simulink model "test_quadcopter"  (R2021b)
settings: Solver=ode45  StartTime=0.0  StopTime=300  FixedStep=Ts  MaxStep=0.001  RelTol=1e-3  AbsTol=1e-3
model workspace (MATLAB code in the model file):
  | load('xy_data_membrane.mat');
undefined symbols (not defined in the file): kd_altitude, kd_attitude, kd_position, ki_altitude, ki_attitude, kp_altitude, kp_attitude, kp_position, propeller, X, x0, xrot, Y, y0, yrot, Z, z0, zrot
libraries: sm_lib x83, fl_lib x40, nesl_utility x34, aerolibwind2 x6, slpidlib x4
(part 1 of 4)
settings Model: Creator=The MathWorks, Inc.  LastModifiedBy=tejaswi
settings SolverCC: AutoScaleAbsTol=off  ZeroCrossAlgorithm=Adaptive  AlgebraicLoopSolver=TrustRegion  SolverResetMethod=Robust
settings DataIOCC: ReturnWorkspaceOutputs=off  SignalLoggingName=logsout_sm_quadcopter
settings DebuggingCC: IgnoredZcDiagnostic=none  SFMachineParentedDataDiag=warning
settings SimscapeCC: SimscapeLogType=all  SimscapeLogSimulationStatistics=on  SimscapeLogName=simlog_sm_quadcopter  SimscapeLogLimitData=off
settings DiagnosticsConfigSet: SimMechanicsRigidlyBoundBlock=none
settings ExplorerConfigSet: InternalSimMechanicsExplorerSettings="<ExplorerConfiguration><canonicalview>default</canonicalview><AnimationSetting><BasePlaybackSpeed>1.0</BasePlaybackSpeed><PlaybackSpeedFactor>1.0</PlaybackSpeedFactor></AnimationSetting><TilePanel><TileInfo><Tiles Columns=\"1\" Count=\"1\" Rows=\"1\"><Column Weight=\"1\"/><Row Weight=\"1\"/><Tile Height=\"1\" Width=\"1\" X=\"0\" Y=\"0\"/></Tiles></TileInfo><SceneInfo><SceneViewer><BGColor><R>0.400000005960464478</R><G>0.800000011920928955</G><B>1</B></BGColor><Camera><DoPerspective>on</DoPerspective><Position><X>-6.15419739613543015e-08</X><Y>-14.2688678910713858</Y><Z>-0.120593802588993895</Z></Position><Center><X>-6.15419739613543015e-08</X><Y>-5.00943414473349335</Y><Z>-0.120593802588992993</Z></Center><Up><X>0</X><Y>-2.49956154589103037e-16</Y><Z>1</Z></Up><ViewLimDist>1</ViewLimDist><YLim>0.466307658154998583</YLim><XLim>0.642537642675115039</XLim></Camera></SceneViewer></SceneInfo></TilePanel><MechEditorPanel><Cameras><Camera><Id>Camera1</Id><Value><Name>Camera1</Name><NativeCamera><PositionKeyframeSet><Keyframe><Time>0</Time><Value><X>-6.1541973961354302e-08</X><Y>-14.268867891071386</Y><Z>-0.1205938025889939</Z></Value></Keyframe><Keyframe><Time>1.9750000000000001</Time><Value><X>0.69357816146467988</X><Y>-14.804552995771699</Y><Z>2.1747680387120214</Z></Value></Keyframe><Keyframe><Time>4.0499999999999998</Time><Value><X>-1.6597740498874662</X><Y>-11.736154408489586</Y><Z>3.2279651603213511</Z></Value></Keyframe><Keyframe><Time>6</Time><Value><X>-1.4506804349012337</X><Y>-10.190737244494224</Y><Z>3.5728880702176977</Z></Value></Keyframe><Keyframe><Time>8</Time><Value><X>-1.6299263783474844</X><Y>-10.672186518254485</Y><Z>3.1366411391344338</Z></Value></Keyframe><Keyframe><Time>10</Time><Value><X>0.18587558187085493</X><Y>-7.6738882503163852</Y><Z>3.8257660713229682</Z></Value></Keyframe><Keyframe><Time>12</Time><Value><X>1.4883977802616708</X><Y>-8.4980171831454285</Y><Z>3.8627593448850166</Z></Value></Keyframe><Keyframe><Time>14</Time><Value><X>1.9893590360011646</X><Y>-6.4957785736357501</Y><Z>3.7251488250353217</Z></Value></Keyframe><Keyframe><Time>16</Time><Value><X>3.6270195589678793</X><Y>-6.36852658984645</Y><Z>3.5837326656674442</Z></Value></Keyframe><Keyframe><Time>18</Time><Value><X>4.1090510945125924</X><Y>-5.5357120217518236</Y><Z>3.2752105329973098</Z></Value></Keyframe><Keyframe><Time>20</Time><Value><X>4.1663622380806169</X><Y>-4.0387452486279827</Y><Z>2.5605170976103575</Z></Value></Keyframe><Keyframe><Time>22</Time><Value><X>4.859351912085474</X><Y>-0.43949351172743789</Y><Z>0.95256853851762346</Z></Value></Keyframe></PositionKeyframeSet><CenterKeyframeSet><Keyframe><Time>0</Time><Value><X>-6.1541973961354302e-08</X><Y>-5.0094341447334934</Y><Z>-0.12059380258899299</Z></Value></Keyframe><Keyframe><Time>1.9750000000000001</Time><Value><X>0.69348438643822474</X><Y>-5.2781774058054065</Y><Z>2.1823800390633106</Z></Value></Keyframe><Keyframe><Time>4.0499999999999998</Time><Value><X>-1.687564798021405</X><Y>-3.7348295538313101</Y><Z>3.2262958119221108</Z></Value></Keyframe><Keyframe><Time>6</Time><Value><X>-1.4797051298603214</X><Y>-2.960851752431255</Y><Z>3.5728880702177048</Z></Value></Keyframe><Keyframe><Time>8</Time><Value><X>-1.5997478000361871</X><Y>-3.1953029757138154</Y><Z>3.1365999604490469</Z></Value></Keyframe><Keyframe><Time>10</Time><Value><X>0.24405104343601497</X><Y>-1.6873776010017201</Y><Z>3.8387300040675179</Z></Value></Keyframe><Keyframe><Time>12</Time><Value><X>1.4806541700514058</X><Y>-2.1382106204808444</Y><Z>3.9209906203717133</Z></Value></Keyframe><Keyframe><Time>14</Time><Value><X>1.9523323695945445</X><Y>-1.1203987104972244</Y><Z>3.7938236446623668</Z></Value></Keyframe><Keyframe><Time>16</Time><Value><X>3.5048147463492194</X><Y>-0.99103496830061388</Y><Z>3.6957539225348288</Z></Value></Keyframe><Keyframe><Time>18</Time><Value><X>3.9997564750585872</X><Y>-0.58040744208225181</Y><Z>3.4078217139748177</Z></Value></Keyframe><Keyframe><Time>20</Time><Value><X>4.1020127201493066</X><Y>0.13918949483856302</Y><Z>2.6890918744946277</Z></Value></Keyframe><Keyframe><Time>22</Time><Value><X>4.822225130199671</X><Y>1.9709872026638768</Y><Z>1.0267504104392398</Z></Value></Keyframe></CenterKeyframeSet><UpVectorKeyframeSet><Keyframe><Time>0</Time><Value><X>0</X><Y>-2.4995615458910304e-16</Y><Z>1</Z></Value></Keyframe><Keyframe><Time>1.9750000000000001</Time><Value><X>7.8655746289375513e-09</X><Y>-0.00079904448954799042</Y><Z>0.99999968076390089</Z></Value></Keyframe><Keyframe><Time>4.0499999999999998</Time><Value><X>-7.2455634795717249e-07</X><Y>0.00020863147757072589</Y><Z>0.99999997823619069</Z></Value></Keyframe><Keyframe><Time>6</Time><Value><X>1.915739347589952e-18</X><Y>-4.771997133902034e-16</Y><Z>1</Z></Value></Keyframe><Keyframe><Time>8</Time><Value><X>-9.4628750535966929e-06</X><Y>5.5456610049874724e-06</Y><Z>0.99999999993984978</Z></Value></Keyframe><Keyframe><Time>10</Time><Value><X>-2.1042002088428629e-05</X><Y>-0.002165314484770997</Y><Z>0.99999765548245956</Z></Value></Keyframe><Keyframe><Time>12</Time><Value><X>-1.2110147359015226e-05</X><Y>-0.0091557703719906611</Y><Z>0.99995808498268568</Z></Value></Keyframe><Keyframe><Time>14</Time><Value><X>1.5974517818876299e-05</X><Y>-0.012774655200305431</Y><Z>0.99991840063543591</Z></Value></Keyframe><Keyframe><Time>16</Time><Value><X>0.00020396676808835565</X><Y>-0.020822355385786397</Y><Z>0.99978317044934573</Z></Value></Keyframe><Keyframe><Time>18</Time><Value><X>0.00034721427582766473</X><Y>-0.026744226999041592</Y><Z>0.99964224888930653</Z></Value></Keyframe><Keyframe><Time>20</Time><Value><X>0.00041919561893311426</X><Y>-0.030753705277349098</Y><Z>0.99952690503395014</Z></Value></Keyframe><Keyframe><Time>22</Time><Value><X>0.00041919561893311751</X><Y>-0.030753705277349306</Y><Z>0.99952690503395003</Z></Value></Keyframe></UpVectorKeyframeSet></NativeCamera></Value></Camera></Cameras><GfxPanelCameraMap><MapElement CameraMLId=\"Camera1\" GfxPanelIndex=\"0\"/></GfxPanelCameraMap><VideoCreator><PlaybackSpeedRatio>1.0</PlaybackSpeedRatio><FrameRate>60</FrameRate><VideoFormat>MPEG-4</VideoFormat><FrameSize>[1920 1080]</FrameSize></VideoCreator></MechEditorPanel></ExplorerConfiguration>"

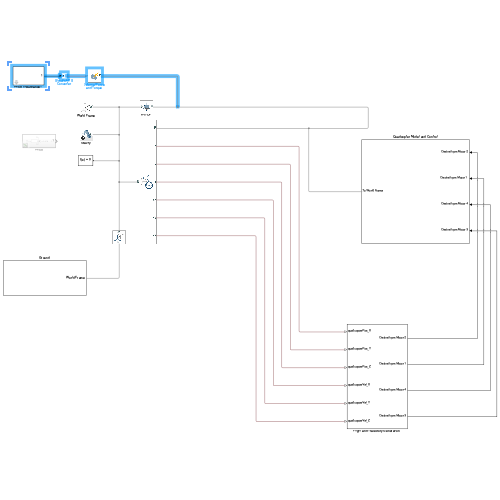
[thumbnail: Simulink's stored preview of the top-level diagram]
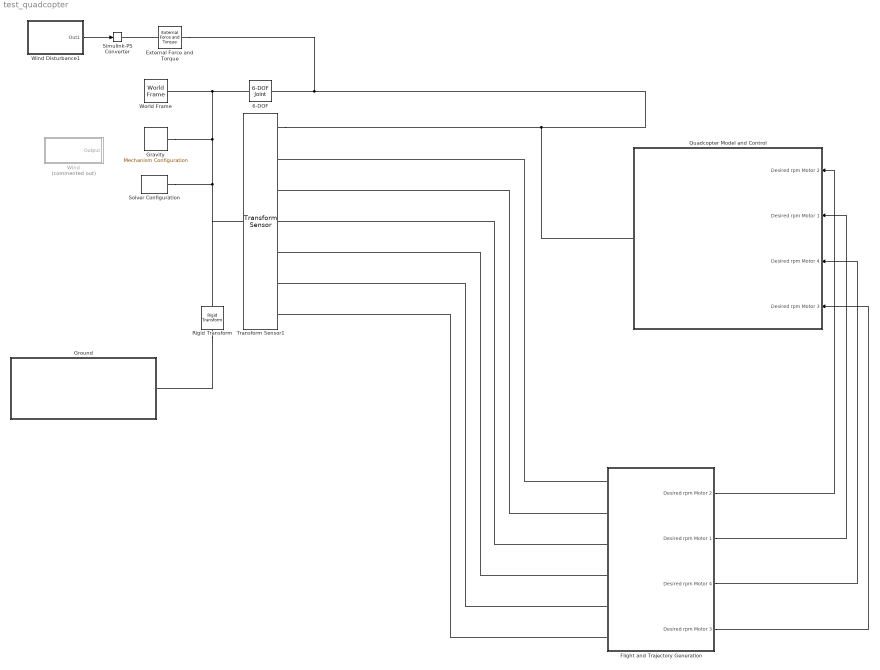
== system test_quadcopter ==
  6-DOF : sm_lib/Joints/6-DOF Joint  JointMode=Normal  SenseConstraintForce=off  SenseConstraintForceX=off  SenseConstraintForceY=off  SenseConstraintForceZ=off  SenseConstraintTorque=off  SenseConstraintTorqueX=off  SenseConstraintTorqueY=off  SenseConstraintTorqueZ=off  SenseTotalForce=off  SenseTotalForceX=off  SenseTotalForceY=off  SenseTotalForceZ=off  SenseTotalTorque=off  SenseTotalTorqueX=off  SenseTotalTorqueY=off  SenseTotalTorqueZ=off  CompositeWrenchDir=FollowerOnBase  CompositeWrenchFrame=BaseFrame  PxEquilibriumPosition=0  PxEquilibriumPositionUnits=m  PxSpringStiffness=0  PxSpringStiffnessUnits=N/m  PxDampingCoefficient=0  PxDampingCoefficientUnits=N/(m/s)  PxTorqueActuationMode=NoTorque  PxMotionActuationMode=ComputedMotion  PxSensePosition=off  PxSenseVelocity=off  PxSenseAcceleration=off  PxSenseTorqueForce=off  PxSenseLowerLimitTorqueForce=off  PxSenseUpperLimitTorqueForce=off  PxLowerLimitSpecify=off  PxLowerLimitBound=-1  PxLowerLimitBoundUnits=m  PxLowerLimitStiffness=1e6  PxLowerLimitStiffnessUnits=N/m  PxLowerLimitDamping=1e3  PxLowerLimitDampingUnits=N/(m/s)  PxLowerLimitTransitionRegionWidth=1e-4  PxLowerLimitTransitionRegionWidthUnits=m  PxUpperLimitSpecify=off  PxUpperLimitBound=1  PxUpperLimitBoundUnits=m  PxUpperLimitStiffness=1e6  PxUpperLimitStiffnessUnits=N/m  PxUpperLimitDamping=1e3  PxUpperLimitDampingUnits=N/(m/s)  PxUpperLimitTransitionRegionWidth=1e-4  PxUpperLimitTransitionRegionWidthUnits=m  PxPositionTargetSpecify=on  PxPositionTargetPriority=High  PxPositionTargetValue=x0  PxPositionTargetValueUnits=m  PxVelocityTargetSpecify=off  PxVelocityTargetPriority=High  PxVelocityTargetValue=0  PxVelocityTargetValueUnits=m/s  PyEquilibriumPosition=0  PyEquilibriumPositionUnits=m  PySpringStiffness=0  PySpringStiffnessUnits=N/m  PyDampingCoefficient=0  PyDampingCoefficientUnits=N/(m/s)  PyTorqueActuationMode=NoTorque  PyMotionActuationMode=ComputedMotion  PySensePosition=off  PySenseVelocity=off  PySenseAcceleration=off  PySenseTorqueForce=off  PySenseLowerLimitTorqueForce=off  PySenseUpperLimitTorqueForce=off  PyLowerLimitSpecify=off  PyLowerLimitBound=-1  PyLowerLimitBoundUnits=m  PyLowerLimitStiffness=1e6  PyLowerLimitStiffnessUnits=N/m  PyLowerLimitDamping=1e3  PyLowerLimitDampingUnits=N/(m/s)  PyLowerLimitTransitionRegionWidth=1e-4  PyLowerLimitTransitionRegionWidthUnits=m  PyUpperLimitSpecify=off  PyUpperLimitBound=1  PyUpperLimitBoundUnits=m  PyUpperLimitStiffness=1e6  PyUpperLimitStiffnessUnits=N/m  PyUpperLimitDamping=1e3  PyUpperLimitDampingUnits=N/(m/s)  PyUpperLimitTransitionRegionWidth=1e-4  PyUpperLimitTransitionRegionWidthUnits=m  PyPositionTargetSpecify=on  PyPositionTargetPriority=High  PyPositionTargetValue=y0  PyPositionTargetValueUnits=m  PyVelocityTargetSpecify=off  PyVelocityTargetPriority=High  PyVelocityTargetValue=0  PyVelocityTargetValueUnits=m/s  PzEquilibriumPosition=0  PzEquilibriumPositionUnits=m  PzSpringStiffness=0  PzSpringStiffnessUnits=N/m  PzDampingCoefficient=0  PzDampingCoefficientUnits=N/(m/s)  PzTorqueActuationMode=NoTorque  PzMotionActuationMode=ComputedMotion  PzSensePosition=off  PzSenseVelocity=off  PzSenseAcceleration=off  PzSenseTorqueForce=off  PzSenseLowerLimitTorqueForce=off  PzSenseUpperLimitTorqueForce=off  PzLowerLimitSpecify=off  PzLowerLimitBound=-1  PzLowerLimitBoundUnits=m  PzLowerLimitStiffness=1e6  PzLowerLimitStiffnessUnits=N/m  PzLowerLimitDamping=1e3  PzLowerLimitDampingUnits=N/(m/s)  PzLowerLimitTransitionRegionWidth=1e-4  PzLowerLimitTransitionRegionWidthUnits=m  PzUpperLimitSpecify=off  PzUpperLimitBound=1  PzUpperLimitBoundUnits=m  PzUpperLimitStiffness=1e6  PzUpperLimitStiffnessUnits=N/m  PzUpperLimitDamping=1e3  PzUpperLimitDampingUnits=N/(m/s)  PzUpperLimitTransitionRegionWidth=1e-4  PzUpperLimitTransitionRegionWidthUnits=m  PzPositionTargetSpecify=on  PzPositionTargetPriority=High  PzPositionTargetValue=z0  PzPositionTargetValueUnits=m  PzVelocityTargetSpecify=off  PzVelocityTargetPriority=High  PzVelocityTargetValue=0  PzVelocityTargetValueUnits=m/s  SphDefPosRotationMethod=None  SphDefPosRotationAngleUnits=deg  SphDefPosRotationStandardAxis=+Z  SphDefPosRotationAngle=0.0  SphDefPosRotationArbitraryAxis=[0 0 1]  SphDefPosFollAlignAxisA=+X  SphDefPosBaseAlignAxisA=+Y  SphDefPosFollAlignAxisB=+Y  SphDefPosBaseAlignAxisB=+Z  SphDefPosRotationSequenceAxes=FollowerAxes  SphDefPosRotationSequence=XYX  SphDefPosRotationSequenceAngles=[0 0 0]  SphDefPosRotationSequenceAnglesUnits=deg  SphDefPosRotationMatrix=[1 0 0; 0 1 0; 0 0 1]  SphEqPosRotationMethod=None  SphEqPosRotationAngleUnits=deg  SphEqPosRotationStandardAxis=+Z  SphEqPosRotationAngle=0.0  SphEqPosRotationArbitraryAxis=[0 0 1]  SphEqPosFollAlignAxisA=+X  SphEqPosBaseAlignAxisA=+Y  SphEqPosFollAlignAxisB=+Y  SphEqPosBaseAlignAxisB=+Z  SphEqPosRotationSequenceAxes=FollowerAxes  SphEqPosRotationSequence=XYX  SphEqPosRotationSequenceAngles=[0 0 0]  SphEqPosRotationSequenceAnglesUnits=deg  SphEqPosRotationMatrix=[1 0 0; 0 1 0; 0 0 1]  SphSpringStiffness=0  SphSpringStiffnessUnits=N*m/deg  SphDampingCoefficient=0  SphDampingCoefficientUnits=N*m/(deg/s)  SphActuateTorqueX=off  SphActuateTorqueY=off  SphActuateTorqueZ=off  SphActuateTorque=off  SphTorqueActuationMode=NoTorque  SphMotionActuationMode=ComputedMotion  SphActuationFrame=BaseFrame  SphSensePosition=off  SphSenseVelocityX=off  SphSenseVelocityY=off  SphSenseVelocityZ=off  SphSenseVelocity=off  SphSenseAccelerationX=off  SphSenseAccelerationY=off  SphSenseAccelerationZ=off  SphSenseAcceleration=off  SphSenseTorqueX=off  SphSenseTorqueY=off  SphSenseTorqueZ=off  SphSenseTorqueForce=off  SphSenseLowerLimitTorqueMag=off  SphSenseUpperLimitTorqueMag=off  SphSensingFrame=BaseFrame  SphLowerLimitSpecify=off  SphLowerLimitBound=15  SphLowerLimitBoundUnits=deg  SphLowerLimitStiffness=1e4  SphLowerLimitStiffnessUnits=N*m/deg  SphLowerLimitDamping=10  SphLowerLimitDampingUnits=N*m/(deg/s)  SphLowerLimitTransitionRegionWidth=0.1  SphLowerLimitTransitionRegionWidthUnits=deg  SphUpperLimitSpecify=off  SphUpperLimitBound=45  SphUpperLimitBoundUnits=deg  SphUpperLimitStiffness=1e4  SphUpperLimitStiffnessUnits=N*m/deg  SphUpperLimitDamping=10  SphUpperLimitDampingUnits=N*m/(deg/s)  SphUpperLimitTransitionRegionWidth=0.1  SphUpperLimitTransitionRegionWidthUnits=deg  SphPositionTargetRotationMethod=RotationSequence  SphPositionTargetRotationAngleUnits=deg  SphPositionTargetRotationStandardAxis=+Y  SphPositionTargetRotationAngle=0  SphPositionTargetRotationArbitraryAxis=[0 0 1]  SphPositionTargetFollAlignAxisA=+X  SphPositionTargetBaseAlignAxisA=+Y  SphPositionTargetFollAlignAxisB=+Y  SphPositionTargetBaseAlignAxisB=+Z  SphPositionTargetRotationSequenceAxes=FollowerAxes  SphPositionTargetRotationSequence=XYZ  SphPositionTargetRotationSequenceAngles=[xrot yrot zrot]  SphPositionTargetRotationSequenceAnglesUnits=deg  SphPositionTargetRotationMatrix=[1 0 0; 0 1 0; 0 0 1]  SphPositionTargetSpecify=on  SphPositionTargetPriority=High  SphVelocityTargetValue=[0 0 0]  SphVelocityTargetValueUnits=deg/s  SphVelocityTargetSpecify=off  SphVelocityTargetPriority=High  SphVelocityTargetInFollowerFrame=on
  External Force and Torque : sm_lib/Forces and Torques/External Force and Torque  ForceResolutionFrame=World  EnableForceX=off  EnableForceY=off  EnableForceZ=off  EnableForce=on  TorqueResolutionFrame=AttachedFrame  EnableTorqueX=off  EnableTorqueY=off  EnableTorqueZ=off  EnableTorque=off
  "Flight and Trajectory Generation " : Subsystem
  Gravity : sm_lib/Utilities/Mechanism Configuration  UniformGravity=Constant  GravityVector=[0 0 -9.80665]  GravityUnits=m/s^2  LinearizationDelta=0.001  JointModeTransitionNonlinearIterations=2
  Ground : Subsystem
  Quadcopter Model and Control : Subsystem
  Rigid Transform : sm_lib/Frames and Transforms/Rigid Transform  TranslationMethod=StandardAxis  TranslationStandardOffset=0.25  TranslationLengthUnit=m  TranslationStandardAxis=-Z  TranslationCartesianOffset=[0 0 0]  TranslationROffset=0  TranslationROffsetUnits=m  TranslationZOffset=0  TranslationZOffsetUnits=m  TranslationThetaOffset=0  TranslationThetaOffsetUnits=deg  RotationMethod=None  RotationAngleUnits=deg  RotationStandardAxis=+Z  RotationAngle=0.0  RotationArbitraryAxis=[0 0 1]  FollAlignAxisA=+X  BaseAlignAxisA=+Y  FollAlignAxisB=+Y  BaseAlignAxisB=+Z  RotationSequenceAxes=FollowerAxes  RotationSequence=XYX  RotationSequenceAngles=[0 0 0]  RotationSequenceAnglesUnits=deg  RotationMatrix=[1 0 0; 0 1 0; 0 0 1]
  Simulink-PS Converter : nesl_utility/Simulink-PS Converter  PhysicalDomain=network_engine_domain  SubClassName=ps_input  LeftPortType=input  RightPortType=output  PseudoPeriodic=off  Frequencies=[]  NoiseDistribution=none  NoiseParameters=[]  Unit=1  AffineConversion=off  FilteringAndDerivatives=provide  SimscapeFilterOrder=1  InputFilterTimeConstant=0.001  UdotUserProvided=0
      settings: SourceProductBaseCode=PW,SS
  Solver Configuration : nesl_utility/Solver Configuration  PhysicalDomain=network_engine_domain  SubClassName=solver  LeftPortType=input  RightPortType=generic  Tones=[]  Harmonics=[]  SimulateNoise=off  Profile=off  UseLocalSampling=off  EnableSwitchedLinearOptims=on  FrequencyDomain=off  UseCCode=off  RelTol=0.001  AbsTol=1e-06  MinStep=1e-09  ToWorkspace=off  RevertToSquareIcSolve=off  NumHomotopyIterations=100  PhasorMode=off  PhasorModeNumHarmonics=1  DoDC=off  ResidualTolerance=1e-09  UseLocalSolver=off  LocalSolverChoice=NE_BACKWARD_EULER_ADVANCER  LocalSolverSampleTime=Ts  DoFixedCost=off  MaxNonlinIter=3  MaxModeIter=2  ComputeImpulses=off  ImpulseIterations=2  LinearAlgebra=auto  EquationFormulation=NE_TIME_EF  DelaysMemoryBudget=1024  AutomaticFiltering=on  FilteringTimeConstant=0.001  PartitionStorageMethod=AS_NEEDED  PartitionMemoryBudget=1024  PartitionMethod=ROBUST
      settings: SourceProductBaseCode=PW,SS
  Transform Sensor1 : sm_lib/Frames and Transforms/Transform Sensor  MeasurementFrame=NonRotatingBase  SenseAngle=off  SenseAxis=off  SenseAngle1=off  SenseAngle2=off  SenseAngle3=off  SenseQ=off  SenseR=off  SenseOmegaX=off  SenseOmegaY=off  SenseOmegaZ=off  SenseOmega1=off  SenseOmega2=off  SenseOmega3=off  SenseQDot=off  SenseRDot=off  SenseAlphaX=off  SenseAlphaY=off  SenseAlphaZ=off  SenseAlpha1=off  SenseAlpha2=off  SenseAlpha3=off  SenseQDDot=off  SenseRDDot=off  SenseX=on  SenseY=on  SenseZ=on  SenseRad=off  SenseAzim=off  SenseDist=off  SenseInc=off  SenseXDot=on  SenseYDot=on  SenseZDot=on  SenseRadDot=off  SenseAzimDot=off  SenseDistDot=off  SenseIncDot=off  SenseXDDot=off  SenseYDDot=off  SenseZDDot=off  SenseRadDDot=off  SenseAzimDDot=off  SenseDistDDot=off  SenseIncDDot=off
  Wind : Subsystem  Commented=on
  Wind Disturbance1 : Subsystem  mask{hei=3, spd=1, deg=30}
      mask prompts: hei "Altitude at which wind in acting (meters)"; spd "Speed of wind (m/s)"; deg "Direction of wind (0 is wind coming from north)"
  World Frame : sm_lib/Frames and Transforms/World Frame
  wires:
  "Flight and Trajectory Generation "/1(Desired rpm Motor 2) -> Quadcopter Model and Control/1(Desired rpm Motor 2)
  "Flight and Trajectory Generation "/2(Desired rpm Motor 1) -> Quadcopter Model and Control/2("Desired rpm Motor 1 ")
  "Flight and Trajectory Generation "/3(Desired rpm Motor 4) -> Quadcopter Model and Control/3(Desired rpm Motor 4)
  "Flight and Trajectory Generation "/4(Desired rpm Motor 3) -> Quadcopter Model and Control/4(Desired rpm Motor 3)
  Wind Disturbance1/1(Out1) -> Simulink-PS Converter/1
  connections:
  Gravity/RConn1 -- Solver Configuration/RConn1 -- Transform Sensor1/LConn1 -- Rigid Transform/LConn1 -- 6-DOF/LConn1 -- World Frame/RConn1
  Transform Sensor1/RConn1 -- External Force and Torque/RConn1 -- 6-DOF/RConn1 -- Quadcopter Model and Control/RConn1
  "Flight and Trajectory Generation "/LConn1 -- Transform Sensor1/RConn2
  "Flight and Trajectory Generation "/LConn2 -- Transform Sensor1/RConn3
  "Flight and Trajectory Generation "/LConn3 -- Transform Sensor1/RConn4
  "Flight and Trajectory Generation "/LConn4 -- Transform Sensor1/RConn5
  "Flight and Trajectory Generation "/LConn5 -- Transform Sensor1/RConn6
  "Flight and Trajectory Generation "/LConn6 -- Transform Sensor1/RConn7
  Rigid Transform/RConn1 -- Ground/RConn1
  External Force and Torque/LConn1 -- Simulink-PS Converter/RConn1

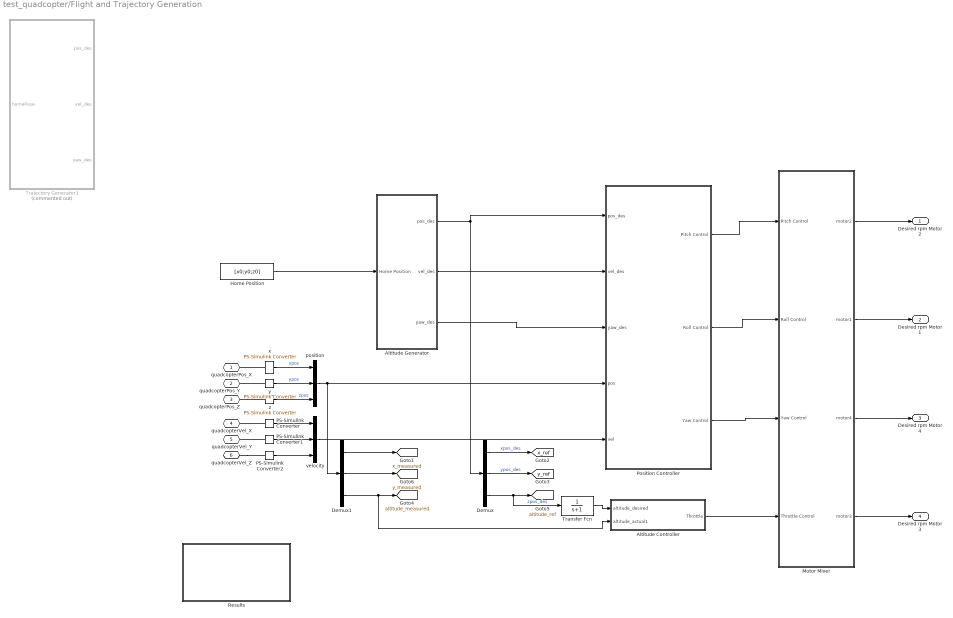
== system test_quadcopter/Flight and Trajectory Generation  ==
  Altitude Controller : Subsystem
  Altitude Generator : Subsystem  mask{alt=5, vel=0}
      mask prompts: alt "Altitude"; vel "Velocity Destination"
  Demux : Demux  Outputs=3
  Demux1 : Demux  Outputs=3
  Home Position : Constant  Value=[x0;y0;z0]
  Motor Mixer : Subsystem
  PS-Simulink Converter : nesl_utility/PS-Simulink Converter  PhysicalDomain=network_engine_domain  SubClassName=ps_output  LeftPortType=input  RightPortType=output  PseudoPeriodic=off  Frequencies=[]  Unit=inherit  AffineConversion=off
      settings: SourceProductBaseCode=PW,SS
  PS-Simulink Converter1 : nesl_utility/PS-Simulink Converter  PhysicalDomain=network_engine_domain  SubClassName=ps_output  LeftPortType=input  RightPortType=output  PseudoPeriodic=off  Frequencies=[]  Unit=inherit  AffineConversion=off
      settings: SourceProductBaseCode=PW,SS
  PS-Simulink Converter2 : nesl_utility/PS-Simulink Converter  PhysicalDomain=network_engine_domain  SubClassName=ps_output  LeftPortType=input  RightPortType=output  PseudoPeriodic=off  Frequencies=[]  Unit=inherit  AffineConversion=off
      settings: SourceProductBaseCode=PW,SS
  Position Controller : Subsystem
  "Results " : Subsystem
  Trajectory Generator1 : MATLAB Function  Commented=on  TreatAsAtomicUnit=on
  Transfer Fcn : TransferFcn  Denominator=[1 1]
  position : Mux  Inputs=3
  velocity : Mux  Inputs=3
  x : nesl_utility/PS-Simulink Converter  PhysicalDomain=network_engine_domain  SubClassName=ps_output  LeftPortType=input  RightPortType=output  PseudoPeriodic=off  Frequencies=[]  Unit=1  AffineConversion=off
      settings: SourceProductBaseCode=PW,SS
  y : nesl_utility/PS-Simulink Converter  PhysicalDomain=network_engine_domain  SubClassName=ps_output  LeftPortType=input  RightPortType=output  PseudoPeriodic=off  Frequencies=[]  Unit=1  AffineConversion=off
      settings: SourceProductBaseCode=PW,SS
  z : nesl_utility/PS-Simulink Converter  PhysicalDomain=network_engine_domain  SubClassName=ps_output  LeftPortType=input  RightPortType=output  PseudoPeriodic=off  Frequencies=[]  Unit=1  AffineConversion=off
      settings: SourceProductBaseCode=PW,SS
  quadcopterPos_X : PMIOPort  Side=Left
  quadcopterPos_Y : PMIOPort  Port=2  Side=Left
  quadcopterPos_Z : PMIOPort  Port=3  Side=Left
  quadcopterVel_X : PMIOPort  Port=4  Side=Left
  quadcopterVel_Y : PMIOPort  Port=5  Side=Left
  quadcopterVel_Z : PMIOPort  Port=6  Side=Left
  Desired rpm Motor 2 : Outport
  Desired rpm Motor 1 : Outport  Port=2
  Desired rpm Motor 4 : Outport  Port=3
  Desired rpm Motor 3 : Outport  Port=4
  tag scope: altitude_measured=global, altitude_ref=global, x_measured=global, x_ref=global, y_measured=global, y_ref=global
  wires:
  z/1 -> position/3  "zpos"
  PS-Simulink Converter1/1 -> velocity/2
  PS-Simulink Converter/1 -> velocity/1
  PS-Simulink Converter2/1 -> velocity/3
  x/1 -> position/1  "xpos"
  position/1 -> Demux1/1, Position Controller/4(pos)
  Demux/2 -> [y_ref]  "ypos_des"
  Demux/1 -> [x_ref]  "xpos_des"
  Demux/3 -> Transfer Fcn/1, [altitude_ref]  "zpos_des"
  y/1 -> position/2  "ypos"
  Demux1/1 -> [x_measured]
  Demux1/3 -> Altitude Controller/2(altitude_actual1), [altitude_measured]
  velocity/1 -> Position Controller/5(vel)
  Motor Mixer/1(motor2) -> Desired rpm Motor 2/1
  Motor Mixer/2(motor1) -> Desired rpm Motor 1/1
  Motor Mixer/3(motor4) -> Desired rpm Motor 4/1
  Motor Mixer/4(motor3) -> Desired rpm Motor 3/1
  Altitude Generator/3(yaw_des) -> Position Controller/3(yaw_des)
  Altitude Generator/2(vel_des) -> Position Controller/2(vel_des)
  Altitude Generator/1(pos_des) -> Position Controller/1(pos_des), Demux/1
  Position Controller/2(Roll Control) -> Motor Mixer/2(Roll Control)
  Position Controller/1(Pitch Control) -> Motor Mixer/1(Pitch Control)
  Position Controller/3(Yaw Control) -> Motor Mixer/3(Yaw Control)
  Altitude Controller/1(Throttle) -> Motor Mixer/4(Throttle Control)
  Transfer Fcn/1 -> Altitude Controller/1(altitude_desired)
  Home Position/1 -> Altitude Generator/1(Home Position)
  Demux1/2 -> [y_measured]
  connections:
  y/LConn1 -- quadcopterPos_Y/RConn1
  x/LConn1 -- quadcopterPos_X/RConn1
  PS-Simulink Converter/LConn1 -- quadcopterVel_X/RConn1
  z/LConn1 -- quadcopterPos_Z/RConn1
  PS-Simulink Converter1/LConn1 -- quadcopterVel_Y/RConn1
  quadcopterVel_Z/RConn1 -- PS-Simulink Converter2/LConn1

== system test_quadcopter/Ground ==
  Ground : sm_lib/Body Elements/Brick Solid  GraphicAmbientColor=[0.15 0.15 0.15 1.0]  BasedOnType=Density  BrickDimensions=[10 10 0.1]  BrickDimensionUnits=m  CenterOfMass=[0 0 0]  CenterOfMassUnits=m  GraphicDiffuseColor=[0.60784316 0.4627451 0.3254902]  Density=1000  DensityUnits=kg/m^3  DoExposeReferenceFrame=on  GraphicEmissiveColor=[0.0 0.0 0.0 1.0]  ExportEntireGeometry=on  SerializedFrames=<Frames><Frame><Id>Frame1</Id><Value><Name>Lp</Name><Origin><Source>GeometricFeature</Source><FeatureName>+z surface</FeatureName></Origin><PrimaryAxis><DefinedDirection>+Z</DefinedDirection><Source>ReferenceFrame</Source><SourceDirection>+Z</SourceDirection><FeatureName></FeatureName></PrimaryAxis><SecondaryAxis><DefinedDirection>+X</DefinedDirection><Source>ReferenceFrame</Source><SourceDirection>+X</SourceDirection><FeatureName></FeatureName></SecondaryAxis></Value></Frame></Frames>  MarkerShape=Sphere  MarkerSize=10  GraphicType=FromGeometry  InertiaType=CalculateFromGeometry  Mass=1  MassUnits=kg  MomentsOfInertia=[1 1 1]  MomentsOfInertiaUnits=kg*m^2  GraphicOpacity=1  ProductsOfInertia=[0 0 0]  ProductsOfInertiaUnits=kg*m^2  GraphicShininess=75  GraphicSpecularColor=[0.5 0.5 0.5 1.0]  GraphicVisPropType=SimpleVisualProperties
  World Frame : PMIOPort  Side=Right
  connections:
  World Frame/RConn1 -- Ground/RConn1

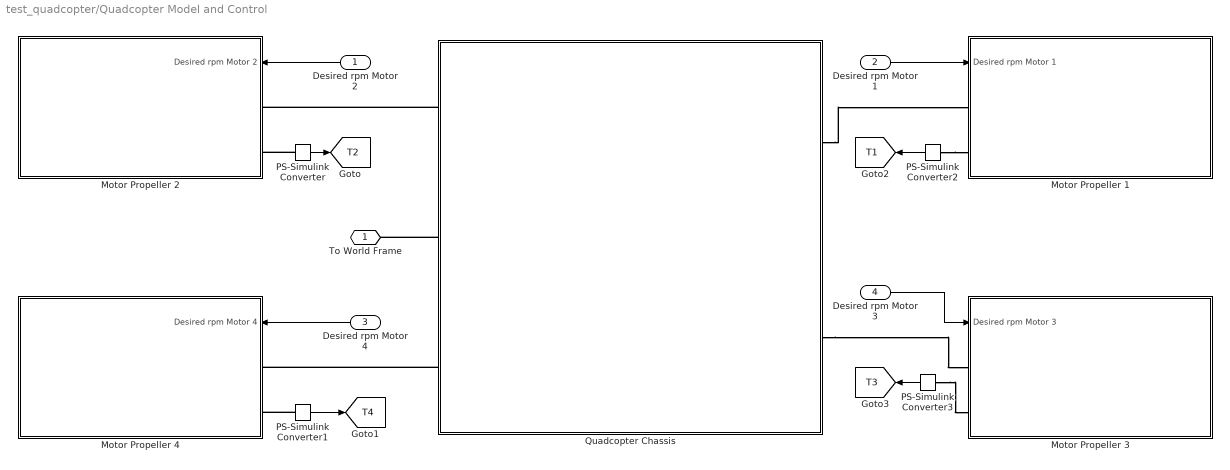
== system test_quadcopter/Quadcopter Model and Control ==
  Desired rpm Motor 2 : Inport
  "Desired rpm Motor 1 " : Inport  Port=2
  Desired rpm Motor 4 : Inport  Port=3
  Desired rpm Motor 3 : Inport  Port=4
  Motor Propeller 1 : Subsystem
  Motor Propeller 2 : Subsystem
  "Motor Propeller 3 " : Subsystem
  Motor Propeller 4 : Subsystem
  PS-Simulink Converter{,1..3} (4 alike) : nesl_utility/PS-Simulink Converter  PhysicalDomain=network_engine_domain  SubClassName=ps_output  LeftPortType=input  RightPortType=output  PseudoPeriodic=off  Frequencies=[]  Unit=inherit  AffineConversion=off
      settings: SourceProductBaseCode=PW,SS
  Quadcopter Chassis : Subsystem
  To World Frame : PMIOPort  Side=Right
  tag scope: T1=global, T2=global, T3=global, T4=global
  wires:
  PS-Simulink Converter/1 -> [T2]
  PS-Simulink Converter1/1 -> [T4]
  PS-Simulink Converter2/1 -> [T1]
  PS-Simulink Converter3/1 -> [T3]
  Desired rpm Motor 2/1 -> Motor Propeller 2/1(Desired rpm Motor 2)
  "Desired rpm Motor 1 "/1 -> Motor Propeller 1/1(Desired rpm Motor 1)
  Desired rpm Motor 4/1 -> Motor Propeller 4/1(Desired rpm Motor 4)
  Desired rpm Motor 3/1 -> "Motor Propeller 3 "/1(Desired rpm Motor 3)
  connections:
  Quadcopter Chassis/LConn2 -- To World Frame/RConn1
  Quadcopter Chassis/LConn1 -- Motor Propeller 2/LConn1
  Quadcopter Chassis/RConn1 -- Motor Propeller 1/LConn1
  Quadcopter Chassis/LConn3 -- Motor Propeller 4/LConn1
  PS-Simulink Converter/LConn1 -- Motor Propeller 2/LConn2
  PS-Simulink Converter1/LConn1 -- Motor Propeller 4/LConn2
  PS-Simulink Converter2/LConn1 -- Motor Propeller 1/LConn2
  PS-Simulink Converter3/LConn1 -- "Motor Propeller 3 "/LConn2
  Quadcopter Chassis/RConn2 -- "Motor Propeller 3 "/LConn1

== system test_quadcopter/Wind ==
  Air Cross Sec-Area : Constant
  Air Density : Constant  Value=1.299
  External Force and Torque : sm_lib/Forces and Torques/External Force and Torque  ForceResolutionFrame=World  EnableForceX=off  EnableForceY=off  EnableForceZ=off  EnableForce=on  TorqueResolutionFrame=AttachedFrame  EnableTorqueX=off  EnableTorqueY=off  EnableTorqueZ=off  EnableTorque=off
  Horizontal Wind Model : aerolibwind2/Horizontal Wind Model  units=Metric (MKS)  Vw_source=Internal  Vwind=0.7  W_source=Internal  Wdeg=0
      settings: SourceProductBaseCode=AE
  IdentityMatrix : IdentityMatrix  OutputDimensions=3
  Product : Product  Inputs=3
  Simulink-PS Converter : nesl_utility/Simulink-PS Converter  PhysicalDomain=network_engine_domain  SubClassName=ps_input  LeftPortType=input  RightPortType=output  PseudoPeriodic=off  Frequencies=[]  NoiseDistribution=none  NoiseParameters=[]  Unit=1  AffineConversion=off  FilteringAndDerivatives=provide  SimscapeFilterOrder=1  InputFilterTimeConstant=0.001  UdotUserProvided=0
      settings: SourceProductBaseCode=PW,SS
  Output : Outport
  wires:
  IdentityMatrix/1 -> Horizontal Wind Model/1
  Product/1 -> Simulink-PS Converter/1
  Air Density/1 -> Product/1
  Horizontal Wind Model/1 -> Product/2
  Air Cross Sec-Area/1 -> Product/3
  connections:
  Simulink-PS Converter/RConn1 -- External Force and Torque/LConn1

== system test_quadcopter/Wind Disturbance1 ==
  Air Cross Sec-Area : Constant
  Air Density : Constant  Value=1.299
  Horizontal Wind Model : aerolibwind2/Horizontal Wind Model  units=Metric (MKS)  Vw_source=Internal  Vwind=spd  W_source=Internal  Wdeg=deg
      settings: SourceProductBaseCode=AE
  Horizontal Wind Model1 : aerolibwind2/Horizontal Wind Model  units=Metric (MKS)  Vw_source=Internal  Vwind=0  W_source=Internal  Wdeg=0
      settings: SourceProductBaseCode=AE
  IdentityMatrix : IdentityMatrix  OutputDimensions=3
  Product : Product  Inputs=3
  Pulse Generator : DiscretePulseGenerator  PulseType=Time based  Period=300  PulseWidth=50
  Switch : Switch  Criteria=u2 > Threshold
  Wind Shear Model1 : aerolibwind2/Wind Shear Model  Commented=on  units=Metric (MKS)  phase=Category C - Terminal Flight Phase  W_20=spd  Wdeg=deg
  Out1 : Outport
  wires:
  Horizontal Wind Model1/1 -> Switch/1
  Pulse Generator/1 -> Switch/2
  Switch/1 -> Product/2
  Product/1 -> Out1/1
  Air Density/1 -> Product/1
  Air Cross Sec-Area/1 -> Product/3
  Horizontal Wind Model/1 -> Switch/3
  IdentityMatrix/1 -> Horizontal Wind Model/1, Horizontal Wind Model1/1

== system test_quadcopter/Flight and Trajectory Generation /Altitude Controller ==
  altitude_desired : Inport
  altitude_actual1 : Inport  Port=2
  Add : Sum  Inputs=+-
  Constant : Constant  Value=2*pi*propeller.hover_speed
  Gain3 : Gain  Gain=2*pi/(0.254^4 * sqrt(1.225))
  PID Controller2 : slpidlib/PID Controller  Controller=PID  Form=Parallel  TimeDomain=Continuous-time  UseExternalTs=off  SampleTime=-1  IntegratorMethod=Forward Euler  FilterMethod=Forward Euler  ControllerParametersSource=internal  P=kp_altitude  I=ki_altitude  D=kd_altitude  UseFilter=on  N=1000  TunerSelectOption=Transfer Function Based (PID Tuner App)  InitialConditionSource=internal  InitialConditionForIntegrator=0  InitialConditionForFilter=0  DifferentiatorICPrevScaledInput=0  ExternalReset=none  TrackingMode=off  Kt=1  LimitOutput=on  SatLimitsSource=internal  UpperSaturationLimit=50  LowerSaturationLimit=-50  LinearizeAsGain=on  AntiWindupMode=none  Kb=1  POutMin=[]  POutMax=[]  IOutMin=[]  IOutMax=[]  DOutMin=[]  DOutMax=[]  NOutMin=[]  NOutMax=[]  SumOutMin=[]  SumOutMax=[]  SaturationOutMin=[]  SaturationOutMax=[]  PParamMin=[]  PParamMax=[]  IParamMin=[]  IParamMax=[]  DParamMin=[]  DParamMax=[]  NParamMin=[]  NParamMax=[]  KbParamMin=[]  KbParamMax=[]  KtParamMin=[]  KtParamMax=[]  KbOutMin=[]  KbOutMax=[]  KtOutMin=[]  KtOutMax=[]  IntegratorOutMin=[]  IntegratorOutMax=[]  FilterOutMin=[]  FilterOutMax=[]  SumI1OutMin=[]  SumI1OutMax=[]  SumI2OutMin=[]  SumI2OutMax=[]  SumI3OutMin=[]  SumI3OutMax=[]  SumI4OutMin=[]  SumI4OutMax=[]  SumDOutMin=[]  SumDOutMax=[]  DifferentiatorOutMin=[]  DifferentiatorOutMax=[]  FilterDiffOutCoefMin=[]  FilterDiffOutCoefMax=[]  ReciprocalOutMin=[]  ReciprocalOutMax=[]  SumDenOutMin=[]  SumDenOutMax=[]  SumNumOutMin=[]  SumNumOutMax=[]  DivideOutMin=[]  DivideOutMax=[]  UdiffTsProdOutMin=[]  UdiffTsProdOutMax=[]  NTsProdOutMin=[]  NTsProdOutMax=[]  UintegralTsProdOutMin=[]  UintegralTsProdOutMax=[]  UngainTsProdOutMin=[]  UngainTsProdOutMax=[]  IntegratorContinuousStateAttributes=''  IntegratorStateMustResolveToSignalObject=off  IntegratorRTWStateStorageClass=Auto  FilterContinuousStateAttributes=''  FilterStateMustResolveToSignalObject=off  FilterRTWStateStorageClass=Auto  ParallelPVariant=InternalParameters  IdealPVariant=Disabled  IVariant=InternalParameters  DVariant=InternalParameters  IntegratorVariant=Continuous  SatVariant=Enabled  AWVariant=Passthrough  PCopyVariant=Disabled  TRVariant=Disabled  FdbkBlocksVariant=Forward  IdealPFdbkVariant=Disabled  SatFdbkVariant=Disabled  DerivativeFilterVariant=ContFilter  NVariant=InternalParameters  NCopyVariant=Disabled  FilterICVariant=InternalICsFilter  IntegratorICVariant=InternalICs  ExternalResetVariant=Disabled  TRSumVariant=Passthrough  SumFdbkVariant=Disabled  SumVariant=Sum_PID  TsampFilterVariant=InternalTs  TsampNgainVariant=Passthrough  TsampIntegralVariant=Passthrough  ExternalSaturationOutDataTypeStr=Inherit: Same as second input
  Sum : Sum  Inputs=|++
  Throttle : Outport
  wires:
  Sum/1 -> Throttle/1
  Constant/1 -> Sum/2
  Gain3/1 -> Sum/1
  Add/1 -> PID Controller2/1
  altitude_desired/1 -> Add/1
  altitude_actual1/1 -> Add/2
  PID Controller2/1 -> Gain3/1

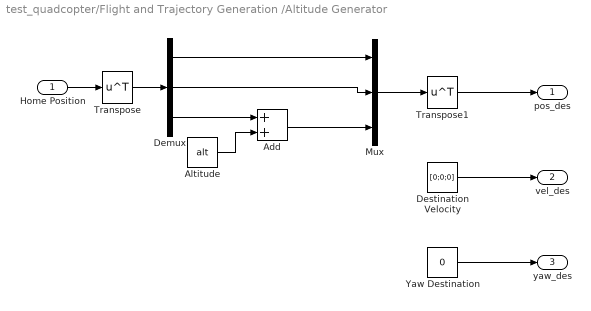
== system test_quadcopter/Flight and Trajectory Generation /Altitude Generator ==
  Home Position : Inport
  Add : Sum
  Altitude : Constant  Value=alt
  Demux : Demux  Outputs=3
  Destination Velocity : Constant  Value=[0;0;0]
  Mux : Mux  Inputs=3
  Transpose : Math  Operator=transpose  SaturateOnIntegerOverflow=on
  Transpose1 : Math  Operator=transpose  SaturateOnIntegerOverflow=on
  Yaw Destination : Constant  Value=0
  pos_des : Outport
  vel_des : Outport  Port=2
  yaw_des : Outport  Port=3
  wires:
  Home Position/1 -> Transpose/1
  Transpose/1 -> Demux/1
  Demux/3 -> Add/1
  Altitude/1 -> Add/2
  Demux/1 -> Mux/1
  Demux/2 -> Mux/2
  Add/1 -> Mux/3
  Mux/1 -> Transpose1/1
  Transpose1/1 -> pos_des/1
  Yaw Destination/1 -> yaw_des/1
  Destination Velocity/1 -> vel_des/1

== system test_quadcopter/Flight and Trajectory Generation /Motor Mixer ==
  Pitch Control : Inport
  Roll Control : Inport  Port=2
  Yaw Control : Inport  Port=3
  Throttle Control : Inport  Port=4
  Add4 : Sum  Inputs=+--+
  Add5 : Sum  Inputs=--++
  Add6 : Sum  Inputs=-+-+
  Add7 : Sum  Inputs=++++
  motor2 : Outport
  motor1 : Outport  Port=2
  motor4 : Outport  Port=3
  motor3 : Outport  Port=4
  wires:
  Add7/1 -> motor3/1
  Add6/1 -> motor4/1
  Add4/1 -> motor1/1
  Add5/1 -> motor2/1
  Roll Control/1 -> Add7/1, Add6/1, Add4/1, Add5/1
  Pitch Control/1 -> Add4/2, Add5/2, Add7/2, Add6/2
  Yaw Control/1 -> Add7/3, Add6/3, Add4/3, Add5/3
  Throttle Control/1 -> Add6/4, Add4/4, Add5/4, Add7/4

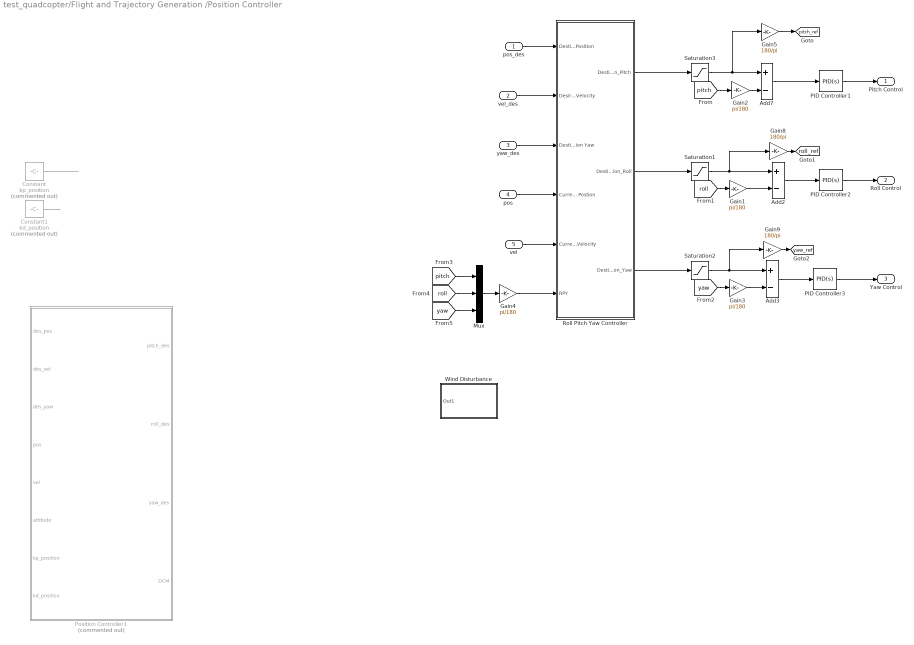
== system test_quadcopter/Flight and Trajectory Generation /Position Controller ==
  pos_des : Inport
  vel_des : Inport  Port=2
  yaw_des : Inport  Port=3
  pos : Inport  Port=4
  vel : Inport  Port=5
  Add2 : Sum  Inputs=+-
  Add3 : Sum  Inputs=+-
  Add7 : Sum  Inputs=+-
  Constant : Constant  Commented=on  Value=kp_position
  Constant1 : Constant  Commented=on  Value=kd_position
  Gain{1..4} (4 alike) : Gain  Gain=pi/180
  Gain5 : Gain  Gain=180/pi
  Gain8 : Gain  Gain=180/pi
  Gain9 : Gain  Gain=180/pi
  Mux : Mux  Inputs=3
  PID Controller1 : slpidlib/PID Controller  Controller=PID  Form=Parallel  TimeDomain=Continuous-time  UseExternalTs=off  SampleTime=-1  IntegratorMethod=Forward Euler  FilterMethod=Forward Euler  ControllerParametersSource=internal  P=kp_attitude  I=ki_attitude  D=kd_attitude  UseFilter=on  N=100  TunerSelectOption=Transfer Function Based (PID Tuner App)  InitialConditionSource=internal  InitialConditionForIntegrator=0  InitialConditionForFilter=0  DifferentiatorICPrevScaledInput=0  ExternalReset=none  TrackingMode=off  Kt=1  LimitOutput=on  SatLimitsSource=internal  UpperSaturationLimit=50  LowerSaturationLimit=-50  LinearizeAsGain=on  AntiWindupMode=none  Kb=1  POutMin=[]  POutMax=[]  IOutMin=[]  IOutMax=[]  DOutMin=[]  DOutMax=[]  NOutMin=[]  NOutMax=[]  SumOutMin=[]  SumOutMax=[]  SaturationOutMin=[]  SaturationOutMax=[]  PParamMin=[]  PParamMax=[]  IParamMin=[]  IParamMax=[]  DParamMin=[]  DParamMax=[]  NParamMin=[]  NParamMax=[]  KbParamMin=[]  KbParamMax=[]  KtParamMin=[]  KtParamMax=[]  KbOutMin=[]  KbOutMax=[]  KtOutMin=[]  KtOutMax=[]  IntegratorOutMin=[]  IntegratorOutMax=[]  FilterOutMin=[]  FilterOutMax=[]  SumI1OutMin=[]  SumI1OutMax=[]  SumI2OutMin=[]  SumI2OutMax=[]  SumI3OutMin=[]  SumI3OutMax=[]  SumI4OutMin=[]  SumI4OutMax=[]  SumDOutMin=[]  SumDOutMax=[]  DifferentiatorOutMin=[]  DifferentiatorOutMax=[]  FilterDiffOutCoefMin=[]  FilterDiffOutCoefMax=[]  ReciprocalOutMin=[]  ReciprocalOutMax=[]  SumDenOutMin=[]  SumDenOutMax=[]  SumNumOutMin=[]  SumNumOutMax=[]  DivideOutMin=[]  DivideOutMax=[]  UdiffTsProdOutMin=[]  UdiffTsProdOutMax=[]  NTsProdOutMin=[]  NTsProdOutMax=[]  UintegralTsProdOutMin=[]  UintegralTsProdOutMax=[]  UngainTsProdOutMin=[]  UngainTsProdOutMax=[]  IntegratorContinuousStateAttributes=''  IntegratorStateMustResolveToSignalObject=off  IntegratorRTWStateStorageClass=Auto  FilterContinuousStateAttributes=''  FilterStateMustResolveToSignalObject=off  FilterRTWStateStorageClass=Auto  ParallelPVariant=InternalParameters  IdealPVariant=Disabled  IVariant=InternalParameters  DVariant=InternalParameters  IntegratorVariant=Continuous  SatVariant=Enabled  AWVariant=Passthrough  PCopyVariant=Disabled  TRVariant=Disabled  FdbkBlocksVariant=Forward  IdealPFdbkVariant=Disabled  SatFdbkVariant=Disabled  DerivativeFilterVariant=ContFilter  NVariant=InternalParameters  NCopyVariant=Disabled  FilterICVariant=InternalICsFilter  IntegratorICVariant=InternalICs  ExternalResetVariant=Disabled  TRSumVariant=Passthrough  SumFdbkVariant=Disabled  SumVariant=Sum_PID  TsampFilterVariant=InternalTs  TsampNgainVariant=Passthrough  TsampIntegralVariant=Passthrough  ExternalSaturationOutDataTypeStr=Inherit: Same as second input
  PID Controller2 : slpidlib/PID Controller  Controller=PID  Form=Parallel  TimeDomain=Continuous-time  UseExternalTs=off  SampleTime=-1  IntegratorMethod=Forward Euler  FilterMethod=Forward Euler  ControllerParametersSource=internal  P=kp_attitude  I=ki_attitude  D=kd_attitude  UseFilter=on  N=100  TunerSelectOption=Transfer Function Based (PID Tuner App)  InitialConditionSource=internal  InitialConditionForIntegrator=0  InitialConditionForFilter=0  DifferentiatorICPrevScaledInput=0  ExternalReset=none  TrackingMode=off  Kt=1  LimitOutput=on  SatLimitsSource=internal  UpperSaturationLimit=50  LowerSaturationLimit=-50  LinearizeAsGain=on  AntiWindupMode=none  Kb=1  POutMin=[]  POutMax=[]  IOutMin=[]  IOutMax=[]  DOutMin=[]  DOutMax=[]  NOutMin=[]  NOutMax=[]  SumOutMin=[]  SumOutMax=[]  SaturationOutMin=[]  SaturationOutMax=[]  PParamMin=[]  PParamMax=[]  IParamMin=[]  IParamMax=[]  DParamMin=[]  DParamMax=[]  NParamMin=[]  NParamMax=[]  KbParamMin=[]  KbParamMax=[]  KtParamMin=[]  KtParamMax=[]  KbOutMin=[]  KbOutMax=[]  KtOutMin=[]  KtOutMax=[]  IntegratorOutMin=[]  IntegratorOutMax=[]  FilterOutMin=[]  FilterOutMax=[]  SumI1OutMin=[]  SumI1OutMax=[]  SumI2OutMin=[]  SumI2OutMax=[]  SumI3OutMin=[]  SumI3OutMax=[]  SumI4OutMin=[]  SumI4OutMax=[]  SumDOutMin=[]  SumDOutMax=[]  DifferentiatorOutMin=[]  DifferentiatorOutMax=[]  FilterDiffOutCoefMin=[]  FilterDiffOutCoefMax=[]  ReciprocalOutMin=[]  ReciprocalOutMax=[]  SumDenOutMin=[]  SumDenOutMax=[]  SumNumOutMin=[]  SumNumOutMax=[]  DivideOutMin=[]  DivideOutMax=[]  UdiffTsProdOutMin=[]  UdiffTsProdOutMax=[]  NTsProdOutMin=[]  NTsProdOutMax=[]  UintegralTsProdOutMin=[]  UintegralTsProdOutMax=[]  UngainTsProdOutMin=[]  UngainTsProdOutMax=[]  IntegratorContinuousStateAttributes=''  IntegratorStateMustResolveToSignalObject=off  IntegratorRTWStateStorageClass=Auto  FilterContinuousStateAttributes=''  FilterStateMustResolveToSignalObject=off  FilterRTWStateStorageClass=Auto  ParallelPVariant=InternalParameters  IdealPVariant=Disabled  IVariant=InternalParameters  DVariant=InternalParameters  IntegratorVariant=Continuous  SatVariant=Enabled  AWVariant=Passthrough  PCopyVariant=Disabled  TRVariant=Disabled  FdbkBlocksVariant=Forward  IdealPFdbkVariant=Disabled  SatFdbkVariant=Disabled  DerivativeFilterVariant=ContFilter  NVariant=InternalParameters  NCopyVariant=Disabled  FilterICVariant=InternalICsFilter  IntegratorICVariant=InternalICs  ExternalResetVariant=Disabled  TRSumVariant=Passthrough  SumFdbkVariant=Disabled  SumVariant=Sum_PID  TsampFilterVariant=InternalTs  TsampNgainVariant=Passthrough  TsampIntegralVariant=Passthrough  ExternalSaturationOutDataTypeStr=Inherit: Same as second input
  PID Controller3 : slpidlib/PID Controller  Controller=PID  Form=Parallel  TimeDomain=Continuous-time  UseExternalTs=off  SampleTime=-1  IntegratorMethod=Forward Euler  FilterMethod=Forward Euler  ControllerParametersSource=internal  P=kp_attitude  I=ki_attitude  D=kd_attitude  UseFilter=on  N=1000  TunerSelectOption=Transfer Function Based (PID Tuner App)  InitialConditionSource=internal  InitialConditionForIntegrator=0  InitialConditionForFilter=0  DifferentiatorICPrevScaledInput=0  ExternalReset=none  TrackingMode=off  Kt=1  LimitOutput=on  SatLimitsSource=internal  UpperSaturationLimit=50  LowerSaturationLimit=-50  LinearizeAsGain=on  AntiWindupMode=none  Kb=1  POutMin=[]  POutMax=[]  IOutMin=[]  IOutMax=[]  DOutMin=[]  DOutMax=[]  NOutMin=[]  NOutMax=[]  SumOutMin=[]  SumOutMax=[]  SaturationOutMin=[]  SaturationOutMax=[]  PParamMin=[]  PParamMax=[]  IParamMin=[]  IParamMax=[]  DParamMin=[]  DParamMax=[]  NParamMin=[]  NParamMax=[]  KbParamMin=[]  KbParamMax=[]  KtParamMin=[]  KtParamMax=[]  KbOutMin=[]  KbOutMax=[]  KtOutMin=[]  KtOutMax=[]  IntegratorOutMin=[]  IntegratorOutMax=[]  FilterOutMin=[]  FilterOutMax=[]  SumI1OutMin=[]  SumI1OutMax=[]  SumI2OutMin=[]  SumI2OutMax=[]  SumI3OutMin=[]  SumI3OutMax=[]  SumI4OutMin=[]  SumI4OutMax=[]  SumDOutMin=[]  SumDOutMax=[]  DifferentiatorOutMin=[]  DifferentiatorOutMax=[]  FilterDiffOutCoefMin=[]  FilterDiffOutCoefMax=[]  ReciprocalOutMin=[]  ReciprocalOutMax=[]  SumDenOutMin=[]  SumDenOutMax=[]  SumNumOutMin=[]  SumNumOutMax=[]  DivideOutMin=[]  DivideOutMax=[]  UdiffTsProdOutMin=[]  UdiffTsProdOutMax=[]  NTsProdOutMin=[]  NTsProdOutMax=[]  UintegralTsProdOutMin=[]  UintegralTsProdOutMax=[]  UngainTsProdOutMin=[]  UngainTsProdOutMax=[]  IntegratorContinuousStateAttributes=''  IntegratorStateMustResolveToSignalObject=off  IntegratorRTWStateStorageClass=Auto  FilterContinuousStateAttributes=''  FilterStateMustResolveToSignalObject=off  FilterRTWStateStorageClass=Auto  ParallelPVariant=InternalParameters  IdealPVariant=Disabled  IVariant=InternalParameters  DVariant=InternalParameters  IntegratorVariant=Continuous  SatVariant=Enabled  AWVariant=Passthrough  PCopyVariant=Disabled  TRVariant=Disabled  FdbkBlocksVariant=Forward  IdealPFdbkVariant=Disabled  SatFdbkVariant=Disabled  DerivativeFilterVariant=ContFilter  NVariant=InternalParameters  NCopyVariant=Disabled  FilterICVariant=InternalICsFilter  IntegratorICVariant=InternalICs  ExternalResetVariant=Disabled  TRSumVariant=Passthrough  SumFdbkVariant=Disabled  SumVariant=Sum_PID  TsampFilterVariant=InternalTs  TsampNgainVariant=Passthrough  TsampIntegralVariant=Passthrough  ExternalSaturationOutDataTypeStr=Inherit: Same as second input
  Position Controller1 : MATLAB Function  Commented=on  TreatAsAtomicUnit=on
  Roll Pitch Yaw Controller : Subsystem  mask{Kp_pos=0.0175, Kd_pos=0.85}
      mask prompts: Kp_pos "Kp Position"; Kd_pos "Kd Position"
  Saturation1 : Saturate  UpperLimit=pi/3  LowerLimit=-pi/3
  Saturation2 : Saturate  UpperLimit=pi/3  LowerLimit=-pi/3
  Saturation3 : Saturate  UpperLimit=pi/3  LowerLimit=-pi/3
  Wind Disturbance : Subsystem  mask{hei=3, spd=1, deg=30}
      mask prompts: hei "Altitude at which wind in acting (meters)"; spd "Speed of wind (m/s)"; deg "Direction of wind (0 is wind coming from north)"
  Pitch Control : Outport
  Roll Control : Outport  Port=2
  Yaw Control : Outport  Port=3
  tag scope: pitch_ref=global, roll_ref=global, yaw_ref=global
  wires:
  pos/1 -> Roll Pitch Yaw Controller/4(Current Postion)
  pos_des/1 -> Roll Pitch Yaw Controller/1(Destination Position)
  Roll Pitch Yaw Controller/2(Destination_Roll) -> Saturation1/1
  Saturation2/1 -> Gain9/1, Add3/1
  yaw_des/1 -> Roll Pitch Yaw Controller/3(Destination Yaw)
  [yaw] -> Gain3/1
  [roll] -> Gain1/1
  [pitch] -> Gain2/1
  vel_des/1 -> Roll Pitch Yaw Controller/2(Desired Velocity)
  Saturation1/1 -> Gain8/1, Add2/1
  Saturation3/1 -> Add7/1, Gain5/1
  Roll Pitch Yaw Controller/1(Destination_Pitch) -> Saturation3/1
  Mux/1 -> Gain4/1
  [yaw] -> Mux/3
  Gain4/1 -> Roll Pitch Yaw Controller/6(RPY)
  Gain1/1 -> Add2/2
  Gain3/1 -> Add3/2
  Gain5/1 -> [pitch_ref]
  Gain8/1 -> [roll_ref]
  Gain9/1 -> [yaw_ref]
  Gain2/1 -> Add7/2
  Add7/1 -> PID Controller1/1
  PID Controller1/1 -> Pitch Control/1
  Add2/1 -> PID Controller2/1
  PID Controller2/1 -> Roll Control/1
  Add3/1 -> PID Controller3/1
  Constant/1 -> ?
  Constant1/1 -> ?
  Roll Pitch Yaw Controller/3(Destionation_Yaw) -> Saturation2/1
  PID Controller3/1 -> Yaw Control/1
  vel/1 -> Roll Pitch Yaw Controller/5(Current Velocity)
  [pitch] -> Mux/1
  [roll] -> Mux/2

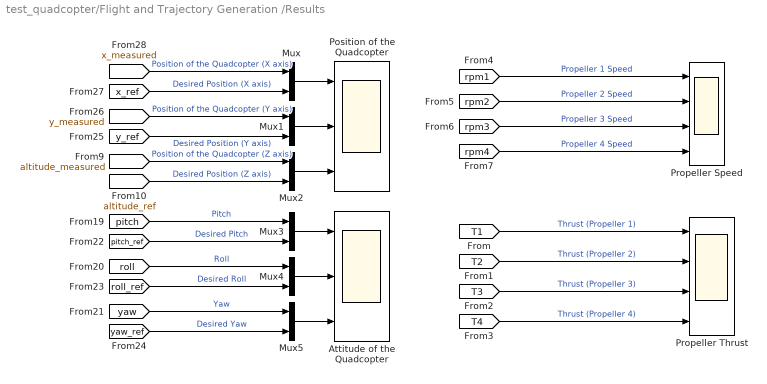
== system test_quadcopter/Flight and Trajectory Generation /Results  ==
  Attitude of the Quadcopter : Scope  NumInputPorts=3
  Mux{,1..5} (6 alike) : Mux  Inputs=2
  Position of the Quadcopter : Scope  NumInputPorts=3
  Propeller Speed : Scope  NumInputPorts=4
  Propeller Thrust : Scope  NumInputPorts=4
  wires:
  [rpm1] -> Propeller Speed/1  "Propeller 1 Speed"
  [rpm2] -> Propeller Speed/2  "Propeller 2 Speed"
  [rpm3] -> Propeller Speed/3  "Propeller 3 Speed"
  [rpm4] -> Propeller Speed/4  "Propeller 4 Speed"
  [altitude_ref] -> Mux2/2  "Desired Position (Z axis)"
  [altitude_measured] -> Mux2/1  "Position of the Quadcopter (Z axis)"
  [pitch] -> Mux3/1  "Pitch"
  [roll] -> Mux4/1  "Roll"
  [yaw] -> Mux5/1  "Yaw"
  [pitch_ref] -> Mux3/2  "Desired Pitch"
  [roll_ref] -> Mux4/2  "Desired Roll"
  [yaw_ref] -> Mux5/2  "Desired Yaw"
  [y_ref] -> Mux1/2  "Desired Position (Y axis)"
  [y_measured] -> Mux1/1  "Position of the Quadcopter (Y axis)"
  [x_ref] -> Mux/2  "Desired Position (X axis)"
  [x_measured] -> Mux/1  "Position of the Quadcopter (X axis)"
  Mux1/1 -> Position of the Quadcopter/2
  Mux/1 -> Position of the Quadcopter/1
  Mux2/1 -> Position of the Quadcopter/3
  Mux4/1 -> Attitude of the Quadcopter/2
  Mux3/1 -> Attitude of the Quadcopter/1
  Mux5/1 -> Attitude of the Quadcopter/3
  [T3] -> Propeller Thrust/3  "Thrust (Propeller 3)"
  [T2] -> Propeller Thrust/2  "Thrust (Propeller 2)"
  [T1] -> Propeller Thrust/1  "Thrust (Propeller 1)"
  [T4] -> Propeller Thrust/4  "Thrust (Propeller 4)"
